simulink model "mrefrobotarm_modified_previous_y_previous_u_previous_ref_pert"  (R2018b)
settings: Solver=FixedStepAuto  StartTime=0.0  StopTime=10  RelTol=1e-3  AbsTol=1e-6
undefined symbols (not defined in the file or in its folder): cc, options
libraries: neural x714, simulink x1
(part 9 of 26)

== system mrefrobotarm_modified_previous_y_previous_u_previous_ref_pert/m=0.01 sd =0.01/Layer 3/Delays 1 ==
  "p{3}" : Inport  PortDimensions=30
      mask Display: e = 0.06;c1 = [120 230 180]/255;c2 = ([120 230 180]+0)/(256+128);c3 = ([120 230 180]+128)/(256+128);patch([0 1 1 0],[0 0 1 1],c1);patch([0 1 1 1-e 1-e 0+e],[0 0 1 1-e 0+e 0+e],c2);patch([0 0 1 1-e 0+e 0+e],[0 1 1 1-e 1-e 0+e],c3);plot([0 1 1 0 0],[0 0 1 1 0]);
  mux : Mux  Inputs=1
      mask Display: e = 0.06;c1 = [120 150 230]/255;c2 = ([120 150 230]+0)/383;c3 = ([120 150 230]+128)/383;patch([0 1 1 0],[0 0 1 1],c1);patch([0 1 1 1-e 1-e 0+e],[0 0 1 1-e 0+e 0+e],c2);patch([0 0 1 1-e 0+e 0+e],[0 1 1 1-e 1-e 0+e],c3);plot([0 1 1 0 0],[0 0 1 1 0]);disp('Mux')
  "pd{3,2}" : Outport
      mask Display: e = 0.06;c1 = [120 230 180]/255;c2 = ([120 230 180]+0)/(256+128);c3 = ([120 230 180]+128)/(256+128);patch([0 1 1 0],[0 0 1 1],c1);patch([0 1 1 1-e 1-e 0+e],[0 0 1 1-e 0+e 0+e],c2);patch([0 0 1 1-e 0+e 0+e],[0 1 1 1-e 1-e 0+e],c3);plot([0 1 1 0 0],[0 0 1 1 0]);
  wires:
  "p{3}"/1 -> mux/1
  mux/1 -> "pd{3,2}"/1

== system mrefrobotarm_modified_previous_y_previous_u_previous_ref_pert/m=0.01 sd =0.01/Layer 3/LW{3,2} ==
  "ad{3,2}" : Inport  PortDimensions=30
      mask Display: e = 0.06;c1 = [120 230 180]/255;c2 = ([120 230 180]+0)/(256+128);c3 = ([120 230 180]+128)/(256+128);patch([0 1 1 0],[0 0 1 1],c1);patch([0 1 1 1-e 1-e 0+e],[0 0 1 1-e 0+e 0+e],c2);patch([0 0 1 1-e 0+e 0+e],[0 1 1 1-e 1-e 0+e],c3);plot([0 1 1 0 0],[0 0 1 1 0]);
  "IW{3,2}(1,:)'" : Constant  Value=[0.0028381381201219024745796559727750718593597412109375;-0.00708260609535531389380214051243456196971237659454345703125;-0.00583488335220346855669593111315407440997660160064697265625;0.01020530930108067869943599959015045897103846073150634765625;0.0035026247420214058798937362126935113337822258472442626953125;0.007372665491954556553355626391521582263521850109100341796875;0.0082512842468972780185509918737807311117649078369140625;-0.006754245741655124334046345069282324402593076229095458984375;0.001683452101721956591096063249324288335628807544708251953125;-0.00690829099421421365112561119303791201673448085784912109375;0.01314880348478297822367721892078407108783721923828125;-0.007470263091506845927469715462621024926193058490753173828125;-0.00542419932097103381363201179965471965260803699493408203125;-0.01146260049752216743368382623202705872245132923126220703125;-0.009116602607925426704493787610772415064275264739990234375;-0.0032803912590090062058323372440327148069627583026885986328125;-0.006661633151908582205213971150215002126060426235198974609375;-0.0289839272926558366716420778175233863294124603271484375;0.007080157965975715332607176577539576101116836071014404296875;1.106395796742202453089021219057030975818634033203125;0.0098157682894019597508172836342055234126746654510498046875;-0.00914110666628639191577665457089096889831125736236572265625;-0.00060787204210546621867272687467220748658291995525360107421875;-0.00883143986489790498717322719812727882526814937591552734375;0.0082676478536601351321255748416660935617983341217041015625;-0.00932936505581516591079083156046181102283298969268798828125;-0.00127195106162408637373584241458956967107951641082763671875;-0.00692592170297301294723535391995028476230800151824951171875;0.009542106880190574791367197349245543591678142547607421875;-0.00879287702148130560775296515885202097706496715545654296875]
      mask Display: e = 0.06;c1 = [120 150 230]/255;c2 = ([120 150 230]+0)/383;c3 = ([120 150 230]+128)/383;patch([0 1 1 0],[0 0 1 1],c1);patch([0 1 1 1-e 1-e 0+e],[0 0 1 1-e 0+e 0+e],c2);patch([0 0 1 1-e 0+e 0+e],[0 1 1 1-e 1-e 0+e],c3);plot([0 1 1 0 0],[0 0 1 1 0]);disp('weights');
  Mux : Mux  Inputs=1
      mask Display: e = 0.06;c1 = [120 150 230]/255;c2 = ([120 150 230]+0)/383;c3 = ([120 150 230]+128)/383;patch([0 1 1 0],[0 0 1 1],c1);patch([0 1 1 1-e 1-e 0+e],[0 0 1 1-e 0+e 0+e],c2);patch([0 0 1 1-e 0+e 0+e],[0 1 1 1-e 1-e 0+e],c3);plot([0 1 1 0 0],[0 0 1 1 0]);disp('Mux');
  dotprod1 : neural/Weight Functions/dotprod
  "lz{3,2}" : Outport
      mask Display: e = 0.06;c1 = [120 230 180]/255;c2 = ([120 230 180]+0)/(256+128);c3 = ([120 230 180]+128)/(256+128);patch([0 1 1 0],[0 0 1 1],c1);patch([0 1 1 1-e 1-e 0+e],[0 0 1 1-e 0+e 0+e],c2);patch([0 0 1 1-e 0+e 0+e],[0 1 1 1-e 1-e 0+e],c3);plot([0 1 1 0 0],[0 0 1 1 0]);
  wires:
  "IW{3,2}(1,:)'"/1 -> dotprod1/1
  "ad{3,2}"/1 -> dotprod1/2
  dotprod1/1 -> Mux/1
  Mux/1 -> "lz{3,2}"/1

== system mrefrobotarm_modified_previous_y_previous_u_previous_ref_pert/m=0.01 sd=0.001/Layer 1/Delays 1 ==
  "p{1}" : Inport  PortDimensions=10
      mask Display: e = 0.06;c1 = [120 230 180]/255;c2 = ([120 230 180]+0)/(256+128);c3 = ([120 230 180]+128)/(256+128);patch([0 1 1 0],[0 0 1 1],c1);patch([0 1 1 1-e 1-e 0+e],[0 0 1 1-e 0+e 0+e],c2);patch([0 0 1 1-e 0+e 0+e],[0 1 1 1-e 1-e 0+e],c3);plot([0 1 1 0 0],[0 0 1 1 0]);
  mux : Mux  Inputs=1
      mask Display: e = 0.06;c1 = [120 150 230]/255;c2 = ([120 150 230]+0)/383;c3 = ([120 150 230]+128)/383;patch([0 1 1 0],[0 0 1 1],c1);patch([0 1 1 1-e 1-e 0+e],[0 0 1 1-e 0+e 0+e],c2);patch([0 0 1 1-e 0+e 0+e],[0 1 1 1-e 1-e 0+e],c3);plot([0 1 1 0 0],[0 0 1 1 0]);disp('Mux')
  "pd{1,1}" : Outport
      mask Display: e = 0.06;c1 = [120 230 180]/255;c2 = ([120 230 180]+0)/(256+128);c3 = ([120 230 180]+128)/(256+128);patch([0 1 1 0],[0 0 1 1],c1);patch([0 1 1 1-e 1-e 0+e],[0 0 1 1-e 0+e 0+e],c2);patch([0 0 1 1-e 0+e 0+e],[0 1 1 1-e 1-e 0+e],c3);plot([0 1 1 0 0],[0 0 1 1 0]);
  wires:
  "p{1}"/1 -> mux/1
  mux/1 -> "pd{1,1}"/1

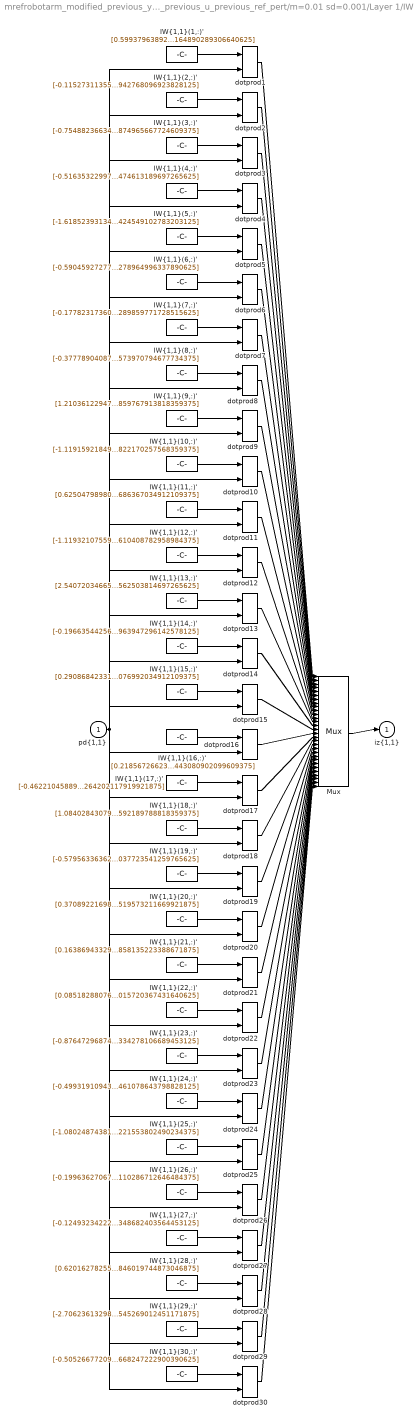
== system mrefrobotarm_modified_previous_y_previous_u_previous_ref_pert/m=0.01 sd=0.001/Layer 1/IW{1,1} ==
  "pd{1,1}" : Inport  PortDimensions=10
      mask Display: e = 0.06;c1 = [120 230 180]/255;c2 = ([120 230 180]+0)/(256+128);c3 = ([120 230 180]+128)/(256+128);patch([0 1 1 0],[0 0 1 1],c1);patch([0 1 1 1-e 1-e 0+e],[0 0 1 1-e 0+e 0+e],c2);patch([0 0 1 1-e 0+e 0+e],[0 1 1 1-e 1-e 0+e],c3);plot([0 1 1 0 0],[0 0 1 1 0]);
  "IW{1,1}(1,:)'" : Constant  Value=[0.59937963892562773349226290520164184272289276123046875;-0.396110549269906020430909165952471084892749786376953125;0.052609198895614932289799270392904873006045818328857421875;0.2316537316693900450115251032912055961787700653076171875;0.1524112985453686397452344181147054769098758697509765625;1.3349014602446771515786849704454652965068817138671875;-1.1072929840932717038270993725745938718318939208984375;0.5612431255418648401445125273312442004680633544921875;1.754962594866394720583002708735875785350799560546875;-0.7339839571900059755904521807678975164890289306640625]
      mask Display: e = 0.06;c1 = [120 150 230]/255;c2 = ([120 150 230]+0)/383;c3 = ([120 150 230]+128)/383;patch([0 1 1 0],[0 0 1 1],c1);patch([0 1 1 1-e 1-e 0+e],[0 0 1 1-e 0+e 0+e],c2);patch([0 0 1 1-e 0+e 0+e],[0 1 1 1-e 1-e 0+e],c3);plot([0 1 1 0 0],[0 0 1 1 0]);disp('Weights');
  "IW{1,1}(10,:)'" : Constant  Value=[-1.1191592184986463021090230540721677243709564208984375;0.486437593586613148399777628583251498639583587646484375;-0.2381955774681704662842918196474784053862094879150390625;-0.1603252511560420423553097180047188885509967803955078125;0.7021448810400536810760740991099737584590911865234375;-0.3126747431395717757851571150240488350391387939453125;0.53741683902639980630056015797890722751617431640625;0.79780181908275016322562578352517448365688323974609375;-0.364527373296976653360701448036707006394863128662109375;-0.7996723179317937191257215090445242822170257568359375]
      mask Display: e = 0.06;c1 = [120 150 230]/255;c2 = ([120 150 230]+0)/383;c3 = ([120 150 230]+128)/383;patch([0 1 1 0],[0 0 1 1],c1);patch([0 1 1 1-e 1-e 0+e],[0 0 1 1-e 0+e 0+e],c2);patch([0 0 1 1-e 0+e 0+e],[0 1 1 1-e 1-e 0+e],c3);plot([0 1 1 0 0],[0 0 1 1 0]);disp('Weights');
  "IW{1,1}(11,:)'" : Constant  Value=[0.62504798980455367196640281690633855760097503662109375;-0.408031907962375317566738885943777859210968017578125;0.501373014961266516564819539780728518962860107421875;0.4833802699139095881974981239181943237781524658203125;-0.362522530256057018416271375826909206807613372802734375;0.2813521372804477227447250697878189384937286376953125;0.8862870179180950547248585280613042414188385009765625;-1.4633494351540063949101977414102293550968170166015625;-0.8590052367755502960022795377881266176700592041015625;0.136037007850934477115600884644663892686367034912109375]
      mask Display: e = 0.06;c1 = [120 150 230]/255;c2 = ([120 150 230]+0)/383;c3 = ([120 150 230]+128)/383;patch([0 1 1 0],[0 0 1 1],c1);patch([0 1 1 1-e 1-e 0+e],[0 0 1 1-e 0+e 0+e],c2);patch([0 0 1 1-e 0+e 0+e],[0 1 1 1-e 1-e 0+e],c3);plot([0 1 1 0 0],[0 0 1 1 0]);disp('Weights');
  "IW{1,1}(12,:)'" : Constant  Value=[-1.119321075598907366810408348101191222667694091796875;-0.171441423142051962980048074314254336059093475341796875;0.980850911593684759992584076826460659503936767578125;0.3269671045177842128026668433449231088161468505859375;0.53034563893542718826523696407093666493892669677734375;-0.54427113197092236163143752492032945156097412109375;-0.74693143368845282825674303239793516695499420166015625;0.1287694280211927055912468631504452787339687347412109375;1.6486561129395822522525349995703436434268951416015625;1.0686346905333097279111598254530690610408782958984375]
      mask Display: e = 0.06;c1 = [120 150 230]/255;c2 = ([120 150 230]+0)/383;c3 = ([120 150 230]+128)/383;patch([0 1 1 0],[0 0 1 1],c1);patch([0 1 1 1-e 1-e 0+e],[0 0 1 1-e 0+e 0+e],c2);patch([0 0 1 1-e 0+e 0+e],[0 1 1 1-e 1-e 0+e],c3);plot([0 1 1 0 0],[0 0 1 1 0]);disp('Weights');
  "IW{1,1}(13,:)'" : Constant  Value=[2.5407203466529697521991693065501749515533447265625;-2.261223662409907131376485267537645995616912841796875;-0.365069530662350316685405005046050064265727996826171875;-0.1886766043105331525087109412197605706751346588134765625;0.0417142901719788350423101519481861032545566558837890625;0.480779756856362094907808568677864968776702880859375;-0.8817579284910894710236561877536587417125701904296875;0.0282120041976467554600827014610331389121711254119873046875;-1.2812114145188753244752888349466957151889801025390625;0.76789716007406616515851283111260272562503814697265625]
      mask Display: e = 0.06;c1 = [120 150 230]/255;c2 = ([120 150 230]+0)/383;c3 = ([120 150 230]+128)/383;patch([0 1 1 0],[0 0 1 1],c1);patch([0 1 1 1-e 1-e 0+e],[0 0 1 1-e 0+e 0+e],c2);patch([0 0 1 1-e 0+e 0+e],[0 1 1 1-e 1-e 0+e],c3);plot([0 1 1 0 0],[0 0 1 1 0]);disp('Weights');
  "IW{1,1}(14,:)'" : Constant  Value=[-0.196635442564636775397701740075717680156230926513671875;0.753137183083409933459506646613590419292449951171875;-0.5846087516227012059744083671830594539642333984375;0.0066653128689167229214973531270516104996204376220703125;0.87919069192101118037641072078258730471134185791015625;-1.478285060894569458156411201343871653079986572265625;1.056716341117762691936832197825424373149871826171875;-0.35476868904702529849970460418262518942356109619140625;-0.5897637965049866703992620386998169124126434326171875;-1.2665284785016901469845151950721628963947296142578125]
      mask Display: e = 0.06;c1 = [120 150 230]/255;c2 = ([120 150 230]+0)/383;c3 = ([120 150 230]+128)/383;patch([0 1 1 0],[0 0 1 1],c1);patch([0 1 1 1-e 1-e 0+e],[0 0 1 1-e 0+e 0+e],c2);patch([0 0 1 1-e 0+e 0+e],[0 1 1 1-e 1-e 0+e],c3);plot([0 1 1 0 0],[0 0 1 1 0]);disp('Weights');
  "IW{1,1}(15,:)'" : Constant  Value=[0.290868423311764157102032868351670913398265838623046875;-1.750593224807010184207456404692493379116058349609375;0.8684408095532607507749389696982689201831817626953125;0.369224320598639355051062693746644072234630584716796875;4.0877592364522090662148912088014185428619384765625;-1.7860833750709534939460354507900774478912353515625;0.274764925669300497101943392408429645001888275146484375;-0.290579497554917853818778894492425024509429931640625;-0.907612828107296376600743315066210925579071044921875;0.046258718737966962597507603049962199293076992034912109375]
      mask Display: e = 0.06;c1 = [120 150 230]/255;c2 = ([120 150 230]+0)/383;c3 = ([120 150 230]+128)/383;patch([0 1 1 0],[0 0 1 1],c1);patch([0 1 1 1-e 1-e 0+e],[0 0 1 1-e 0+e 0+e],c2);patch([0 0 1 1-e 0+e 0+e],[0 1 1 1-e 1-e 0+e],c3);plot([0 1 1 0 0],[0 0 1 1 0]);disp('Weights');
  "IW{1,1}(16,:)'" : Constant  Value=[0.21856726623393207820100769822602160274982452392578125;0.43822988527784667578401922582997940480709075927734375;-0.139288002716730641150633118741097860038280487060546875;0.47802454669038885182175135923898778855800628662109375;-2.458877629721705648790930354152806103229522705078125;0.73280849029216710288636704717646352946758270263671875;0.279458397030770300251134585778345353901386260986328125;0.62598650250979093190295543536194600164890289306640625;1.01423895682535913920219172723591327667236328125;-0.173414588391354873575522788087255321443080902099609375]
      mask Display: e = 0.06;c1 = [120 150 230]/255;c2 = ([120 150 230]+0)/383;c3 = ([120 150 230]+128)/383;patch([0 1 1 0],[0 0 1 1],c1);patch([0 1 1 1-e 1-e 0+e],[0 0 1 1-e 0+e 0+e],c2);patch([0 0 1 1-e 0+e 0+e],[0 1 1 1-e 1-e 0+e],c3);plot([0 1 1 0 0],[0 0 1 1 0]);disp('Weights');
  "IW{1,1}(17,:)'" : Constant  Value=[-0.462210458898908715941189484510687179863452911376953125;0.0562441048399441589911162964199320413172245025634765625;1.6557581521501216759162389280390925705432891845703125;1.4468927892442950966511716615059413015842437744140625;-0.404186313250386841655625858038547448813915252685546875;0.271837747395356765789387054610415361821651458740234375;-1.263092687688632143050426748231984674930572509765625;0.185960700398180633907685432859580032527446746826171875;2.02659382751513650333663463243283331394195556640625;-0.40086308697406003442864630414987914264202117919921875]
      mask Display: e = 0.06;c1 = [120 150 230]/255;c2 = ([120 150 230]+0)/383;c3 = ([120 150 230]+128)/383;patch([0 1 1 0],[0 0 1 1],c1);patch([0 1 1 1-e 1-e 0+e],[0 0 1 1-e 0+e 0+e],c2);patch([0 0 1 1-e 0+e 0+e],[0 1 1 1-e 1-e 0+e],c3);plot([0 1 1 0 0],[0 0 1 1 0]);disp('Weights');
  "IW{1,1}(18,:)'" : Constant  Value=[1.0840284307910679206798931772937066853046417236328125;0.04238645655672386436396692488415283150970935821533203125;0.0647929422435409296809893930912949144840240478515625;-0.2007261202465783489490291913170949555933475494384765625;0.231390749330992295806908032318460755050182342529296875;-0.2493164861823878031277246236641076393425464630126953125;-1.288247138719182061095125391148030757904052734375;0.66489830287387075014038373410585336387157440185546875;-0.87855236053860064071585611600312404334545135498046875;-0.571013622141661070230611585429869592189788818359375]
      mask Display: e = 0.06;c1 = [120 150 230]/255;c2 = ([120 150 230]+0)/383;c3 = ([120 150 230]+128)/383;patch([0 1 1 0],[0 0 1 1],c1);patch([0 1 1 1-e 1-e 0+e],[0 0 1 1-e 0+e 0+e],c2);patch([0 0 1 1-e 0+e 0+e],[0 1 1 1-e 1-e 0+e],c3);plot([0 1 1 0 0],[0 0 1 1 0]);disp('Weights');
  "IW{1,1}(19,:)'" : Constant  Value=[-0.579563363622992877566275637946091592311859130859375;0.0808814352621067544912847324667382054030895233154296875;-0.627693531991440512030067111481912434101104736328125;-0.342503079851861347293606741004623472690582275390625;1.9480020511887434775388783236849121749401092529296875;-1.22709210487031139535929469275288283824920654296875;-1.041532997170801166930687031708657741546630859375;-0.40601996839724840970831110098515637218952178955078125;-0.350497880443465359423527161197853274643421173095703125;0.379106573287681547501648537945584394037723541259765625]
      mask Display: e = 0.06;c1 = [120 150 230]/255;c2 = ([120 150 230]+0)/383;c3 = ([120 150 230]+128)/383;patch([0 1 1 0],[0 0 1 1],c1);patch([0 1 1 1-e 1-e 0+e],[0 0 1 1-e 0+e 0+e],c2);patch([0 0 1 1-e 0+e 0+e],[0 1 1 1-e 1-e 0+e],c3);plot([0 1 1 0 0],[0 0 1 1 0]);disp('Weights');
  "IW{1,1}(2,:)'" : Constant  Value=[-0.11527311355962044370215835442650131881237030029296875;-0.404225992456426597154717228477238677442073822021484375;-0.334837070807286918405765163697651587426662445068359375;0.90518533001313794539299806274357251822948455810546875;2.2543779617530912418033040012232959270477294921875;-2.026726348690087053938668759656138718128204345703125;-0.21181078080885329395499638849287293851375579833984375;-1.79130234483826011882001694175414741039276123046875;1.1268087142547169587913913346710614860057830810546875;-0.97828729118855151103417711055953986942768096923828125]
      mask Display: e = 0.06;c1 = [120 150 230]/255;c2 = ([120 150 230]+0)/383;c3 = ([120 150 230]+128)/383;patch([0 1 1 0],[0 0 1 1],c1);patch([0 1 1 1-e 1-e 0+e],[0 0 1 1-e 0+e 0+e],c2);patch([0 0 1 1-e 0+e 0+e],[0 1 1 1-e 1-e 0+e],c3);plot([0 1 1 0 0],[0 0 1 1 0]);disp('Weights');
  "IW{1,1}(20,:)'" : Constant  Value=[0.370892216980794497960260969193768687546253204345703125;1.8302016509147744915964040046674199402332305908203125;-1.8556216709284181209937969470047391951084136962890625;1.655754682395713661691161178168840706348419189453125;-0.74706859881024545444461182341910898685455322265625;0.8604515450150509447979629840119741857051849365234375;-1.802061941623871010875745923840440809726715087890625;0.12266944769845385121431746711095911450684070587158203125;-2.192229171652474661868836847133934497833251953125;0.367378607338902873902242163239861838519573211669921875]
      mask Display: e = 0.06;c1 = [120 150 230]/255;c2 = ([120 150 230]+0)/383;c3 = ([120 150 230]+128)/383;patch([0 1 1 0],[0 0 1 1],c1);patch([0 1 1 1-e 1-e 0+e],[0 0 1 1-e 0+e 0+e],c2);patch([0 0 1 1-e 0+e 0+e],[0 1 1 1-e 1-e 0+e],c3);plot([0 1 1 0 0],[0 0 1 1 0]);disp('Weights');
  "IW{1,1}(21,:)'" : Constant  Value=[0.1638694332917713103459078638479695655405521392822265625;-0.302284193263745393220887081042747013270854949951171875;-0.385412062490031626094122430004063062369823455810546875;0.8129911212999463288042534259147942066192626953125;-0.85191701402662811659638464334420859813690185546875;-0.53939451890989664750719612129614688456058502197265625;0.441389074698777250649328607323695905506610870361328125;0.5769130466845950877541326917707920074462890625;-1.245667655438771337372827474609948694705963134765625;0.00412112726435204072827911403464895556680858135223388671875]
      mask Display: e = 0.06;c1 = [120 150 230]/255;c2 = ([120 150 230]+0)/383;c3 = ([120 150 230]+128)/383;patch([0 1 1 0],[0 0 1 1],c1);patch([0 1 1 1-e 1-e 0+e],[0 0 1 1-e 0+e 0+e],c2);patch([0 0 1 1-e 0+e 0+e],[0 1 1 1-e 1-e 0+e],c3);plot([0 1 1 0 0],[0 0 1 1 0]);disp('Weights');
  "IW{1,1}(22,:)'" : Constant  Value=[0.08518288076987053092370416607082006521522998809814453125;-0.8537294142013858166961881579481996595859527587890625;0.7741003486488844398394348900183103978633880615234375;0.158479487052409606651082185635459609329700469970703125;-1.6855139048679979030254116878495551645755767822265625;0.2147391184469020775082981344894506037235260009765625;-0.227385538868920378252624914239277131855487823486328125;-0.00452640259162017007110723199048152309842407703399658203125;0.9402929814598015578752665533102117478847503662109375;1.4362169500364247998192013255902566015720367431640625]
      mask Display: e = 0.06;c1 = [120 150 230]/255;c2 = ([120 150 230]+0)/383;c3 = ([120 150 230]+128)/383;patch([0 1 1 0],[0 0 1 1],c1);patch([0 1 1 1-e 1-e 0+e],[0 0 1 1-e 0+e 0+e],c2);patch([0 0 1 1-e 0+e 0+e],[0 1 1 1-e 1-e 0+e],c3);plot([0 1 1 0 0],[0 0 1 1 0]);disp('Weights');
  "IW{1,1}(23,:)'" : Constant  Value=[-0.876472968740060753845000363071449100971221923828125;0.97338759015756204373559512532665394246578216552734375;0.048119337681629716085840442474363953806459903717041015625;0.041438003349266304409237449135616770945489406585693359375;-0.126305138511878689566714228931232355535030364990234375;1.00882944072944980007378035224974155426025390625;-0.93544391369868529206854645963176153600215911865234375;-0.2308533783162892427665013883597566746175289154052734375;-1.6617951684667169320874791083042509853839874267578125;0.07859271650706974032818408204548177309334278106689453125]
      mask Display: e = 0.06;c1 = [120 150 230]/255;c2 = ([120 150 230]+0)/383;c3 = ([120 150 230]+128)/383;patch([0 1 1 0],[0 0 1 1],c1);patch([0 1 1 1-e 1-e 0+e],[0 0 1 1-e 0+e 0+e],c2);patch([0 0 1 1-e 0+e 0+e],[0 1 1 1-e 1-e 0+e],c3);plot([0 1 1 0 0],[0 0 1 1 0]);disp('Weights');
  "IW{1,1}(24,:)'" : Constant  Value=[-0.499319109438899733088845778183895163238048553466796875;0.0249813223099573898655645365352029330097138881683349609375;-0.62391102764310557571292292777798138558864593505859375;0.045969549982219193307031446238397620618343353271484375;0.29761373371729582526512558615650050342082977294921875;0.75652230673170783870062905407394282519817352294921875;-0.21882391321545358042754969574161805212497711181640625;-0.152652868546594489007617312381626106798648834228515625;0.130026205414276230243331156088970601558685302734375;0.210042947632892051945674438684363849461078643798828125]
      mask Display: e = 0.06;c1 = [120 150 230]/255;c2 = ([120 150 230]+0)/383;c3 = ([120 150 230]+128)/383;patch([0 1 1 0],[0 0 1 1],c1);patch([0 1 1 1-e 1-e 0+e],[0 0 1 1-e 0+e 0+e],c2);patch([0 0 1 1-e 0+e 0+e],[0 1 1 1-e 1-e 0+e],c3);plot([0 1 1 0 0],[0 0 1 1 0]);disp('Weights');
  "IW{1,1}(25,:)'" : Constant  Value=[-1.080248743819219203743386970018036663532257080078125;0.90199303598355073940950887845247052609920501708984375;-0.81531722448001942016304610660881735384464263916015625;-0.470572048901045481006377713129040785133838653564453125;-0.215494082328827440964147399427019990980625152587890625;0.73105039783397585129165463513345457613468170166015625;-2.073647250650516138392731591011397540569305419921875;0.0858309743410513303896181014351896010339260101318359375;0.22192825146346584208600916099385358393192291259765625;0.20410220428678493842511443290277384221553802490234375]
      mask Display: e = 0.06;c1 = [120 150 230]/255;c2 = ([120 150 230]+0)/383;c3 = ([120 150 230]+128)/383;patch([0 1 1 0],[0 0 1 1],c1);patch([0 1 1 1-e 1-e 0+e],[0 0 1 1-e 0+e 0+e],c2);patch([0 0 1 1-e 0+e 0+e],[0 1 1 1-e 1-e 0+e],c3);plot([0 1 1 0 0],[0 0 1 1 0]);disp('Weights');
  "IW{1,1}(26,:)'" : Constant  Value=[-0.199636270672255478064727185483206994831562042236328125;0.466242803891780577263403984034084714949131011962890625;-1.786751590761676222740561570390127599239349365234375;0.00230779769893033580296926032815463258884847164154052734375;1.2852038464398283235112785405362956225872039794921875;-1.0973774958082704866768608553684316575527191162109375;0.308005670144092358331278092009597457945346832275390625;-0.35227734504899654854881418941658921539783477783203125;1.0752875894278357549183056107722222805023193359375;-0.38697375163509251105864450437366031110286712646484375]
      mask Display: e = 0.06;c1 = [120 150 230]/255;c2 = ([120 150 230]+0)/383;c3 = ([120 150 230]+128)/383;patch([0 1 1 0],[0 0 1 1],c1);patch([0 1 1 1-e 1-e 0+e],[0 0 1 1-e 0+e 0+e],c2);patch([0 0 1 1-e 0+e 0+e],[0 1 1 1-e 1-e 0+e],c3);plot([0 1 1 0 0],[0 0 1 1 0]);disp('Weights');
  "IW{1,1}(27,:)'" : Constant  Value=[-0.124932342227794979105937045460450462996959686279296875;-0.66631572445832720763547740716603584587574005126953125;-0.02202657447860668915584625437986687757074832916259765625;-0.1792737902950718720251899185313959605991840362548828125;0.4624051360576657554446455833385698497295379638671875;-0.048505735738689235991838444306267774663865566253662109375;0.269052190115036282680449630788643844425678253173828125;0.1233902147738448196179206206579692661762237548828125;0.145988756281055953589742557596764527261257171630859375;0.82365531327662655503019095704075880348682403564453125]
      mask Display: e = 0.06;c1 = [120 150 230]/255;c2 = ([120 150 230]+0)/383;c3 = ([120 150 230]+128)/383;patch([0 1 1 0],[0 0 1 1],c1);patch([0 1 1 1-e 1-e 0+e],[0 0 1 1-e 0+e 0+e],c2);patch([0 0 1 1-e 0+e 0+e],[0 1 1 1-e 1-e 0+e],c3);plot([0 1 1 0 0],[0 0 1 1 0]);disp('Weights');
  "IW{1,1}(28,:)'" : Constant  Value=[0.62016278255009071873615766889997757971286773681640625;0.03190241625757568588728219083350268192589282989501953125;-0.544385606509863340107813201029784977436065673828125;0.1453635890249763418236028655883274041116237640380859375;-0.60065937150521875320663411912391893565654754638671875;-1.1049035559021211927444028333411552011966705322265625;0.312613407122662056991657664184458553791046142578125;0.5588976319380625223942615775740705430507659912109375;-0.93021207078281531455132835617405362427234649658203125;0.74350140785050367053798936467501334846019744873046875]
      mask Display: e = 0.06;c1 = [120 150 230]/255;c2 = ([120 150 230]+0)/383;c3 = ([120 150 230]+128)/383;patch([0 1 1 0],[0 0 1 1],c1);patch([0 1 1 1-e 1-e 0+e],[0 0 1 1-e 0+e 0+e],c2);patch([0 0 1 1-e 0+e 0+e],[0 1 1 1-e 1-e 0+e],c3);plot([0 1 1 0 0],[0 0 1 1 0]);disp('Weights');
  "IW{1,1}(29,:)'" : Constant  Value=[-2.706236132987961173768098888103850185871124267578125;1.605665021864861596867513071629218757152557373046875;0.526580609549972766814107671962119638919830322265625;-0.14272486709085985268075091880746185779571533203125;-1.312819169084094905741721959202550351619720458984375;1.147345692737551825501896018977276980876922607421875;0.410746459531053986768966979070683009922504425048828125;1.2852081431608881612049799514352343976497650146484375;0.1081836722584629539856138080722303129732608795166015625;0.73857624379430841798921392182819545269012451171875]
      mask Display: e = 0.06;c1 = [120 150 230]/255;c2 = ([120 150 230]+0)/383;c3 = ([120 150 230]+128)/383;patch([0 1 1 0],[0 0 1 1],c1);patch([0 1 1 1-e 1-e 0+e],[0 0 1 1-e 0+e 0+e],c2);patch([0 0 1 1-e 0+e 0+e],[0 1 1 1-e 1-e 0+e],c3);plot([0 1 1 0 0],[0 0 1 1 0]);disp('Weights');
  "IW{1,1}(3,:)'" : Constant  Value=[-0.75488236634097571897683565111947245895862579345703125;0.3670412473066251290987338506965897977352142333984375;1.01240774526453236603629193268716335296630859375;0.7161619255534501515825240858248434960842132568359375;0.25623477060716293163267209820332936942577362060546875;1.580258141643140046284088384709320962429046630859375;-0.288265922013249298316850399714894592761993408203125;-0.042314819711078734132403411649647750891745090484619140625;0.5350196659118566788748694307287223637104034423828125;0.3356458871309120350900911944336257874965667724609375]
      mask Display: e = 0.06;c1 = [120 150 230]/255;c2 = ([120 150 230]+0)/383;c3 = ([120 150 230]+128)/383;patch([0 1 1 0],[0 0 1 1],c1);patch([0 1 1 1-e 1-e 0+e],[0 0 1 1-e 0+e 0+e],c2);patch([0 0 1 1-e 0+e 0+e],[0 1 1 1-e 1-e 0+e],c3);plot([0 1 1 0 0],[0 0 1 1 0]);disp('Weights');
  "IW{1,1}(30,:)'" : Constant  Value=[-0.50526677209464765372359806860913522541522979736328125;-0.7086058290307359897042260854505002498626708984375;0.80288187329153604121501075496780686080455780029296875;0.3084326872686131704170975353918038308620452880859375;0.011191847348981577570103951302371569909155368804931640625;-0.13027295381265435736395374988205730915069580078125;-0.63120307203300252130162562025361694395542144775390625;0.59429072606559441016571554428082890808582305908203125;0.98981309673762296608146016296814195811748504638671875;-0.0754501604676642845248579760664142668247222900390625]
      mask Display: e = 0.06;c1 = [120 150 230]/255;c2 = ([120 150 230]+0)/383;c3 = ([120 150 230]+128)/383;patch([0 1 1 0],[0 0 1 1],c1);patch([0 1 1 1-e 1-e 0+e],[0 0 1 1-e 0+e 0+e],c2);patch([0 0 1 1-e 0+e 0+e],[0 1 1 1-e 1-e 0+e],c3);plot([0 1 1 0 0],[0 0 1 1 0]);disp('Weights');
  "IW{1,1}(4,:)'" : Constant  Value=[-0.516353229978596228733067619032226502895355224609375;-1.103631081466493579767984556383453309535980224609375;0.7578291006076636193711237865500152111053466796875;-0.482376012038346624333229328840388916432857513427734375;-1.4371596262453063541641995470854453742504119873046875;-0.1944939411233803927547825196597841568291187286376953125;1.56897655385656431548113687313161790370941162109375;1.288771842824615987410652451217174530029296875;0.0142198876681832973856156598913003108464181423187255859375;0.2646892221021150959359147236682474613189697265625]
      mask Display: e = 0.06;c1 = [120 150 230]/255;c2 = ([120 150 230]+0)/383;c3 = ([120 150 230]+128)/383;patch([0 1 1 0],[0 0 1 1],c1);patch([0 1 1 1-e 1-e 0+e],[0 0 1 1-e 0+e 0+e],c2);patch([0 0 1 1-e 0+e 0+e],[0 1 1 1-e 1-e 0+e],c3);plot([0 1 1 0 0],[0 0 1 1 0]);disp('Weights');
  "IW{1,1}(5,:)'" : Constant  Value=[-1.6185239313409771622076505082077346742153167724609375;0.66121160958456537404259734103106893599033355712890625;0.49893121833904652273616875390871427953243255615234375;-0.0022013083249246136012533536785440446692518889904022216796875;0.33840270003378714047670428044511936604976654052734375;1.8341241878053580194318783469498157501220703125;-1.4131691826434986669625004651607014238834381103515625;0.31651863826449588845690641392138786613941192626953125;0.83507561497049509480206097578047774732112884521484375;-0.2197673461643170622625831356344860978424549102783203125]
      mask Display: e = 0.06;c1 = [120 150 230]/255;c2 = ([120 150 230]+0)/383;c3 = ([120 150 230]+128)/383;patch([0 1 1 0],[0 0 1 1],c1);patch([0 1 1 1-e 1-e 0+e],[0 0 1 1-e 0+e 0+e],c2);patch([0 0 1 1-e 0+e 0+e],[0 1 1 1-e 1-e 0+e],c3);plot([0 1 1 0 0],[0 0 1 1 0]);disp('Weights');
  "IW{1,1}(6,:)'" : Constant  Value=[-0.590459272773774745957098275539465248584747314453125;0.55052745113397139054001172553398646414279937744140625;-0.81263114027772653802372815334820188581943511962890625;-0.43956190723335686332262639552936889231204986572265625;-1.973825194590407949846166957286186516284942626953125;2.03599524499412698474998251185752451419830322265625;-0.335927600637568268826527173587237484753131866455078125;-0.804229659678409536383014710736460983753204345703125;0.0809369564142785602456342530786059796810150146484375;1.1115959245337629912597776637994684278964996337890625]
      mask Display: e = 0.06;c1 = [120 150 230]/255;c2 = ([120 150 230]+0)/383;c3 = ([120 150 230]+128)/383;patch([0 1 1 0],[0 0 1 1],c1);patch([0 1 1 1-e 1-e 0+e],[0 0 1 1-e 0+e 0+e],c2);patch([0 0 1 1-e 0+e 0+e],[0 1 1 1-e 1-e 0+e],c3);plot([0 1 1 0 0],[0 0 1 1 0]);disp('Weights');
  "IW{1,1}(7,:)'" : Constant  Value=[-0.177823173605108630912496892051422037184238433837890625;-0.1643050204328404817477604638042976148426532745361328125;-0.66501256984892875845361004394362680613994598388671875;0.65392664211458717549163566218339838087558746337890625;-1.3627966765753674049932442358112893998622894287109375;0.60552086375707403487211877290974371135234832763671875;0.1617097296379933213383850443278788588941097259521484375;-0.7858432318438748342970256999251432716846466064453125;-0.285345159763251421392027395995683036744594573974609375;-1.1360349772904767551295890370965935289859771728515625]
      mask Display: e = 0.06;c1 = [120 150 230]/255;c2 = ([120 150 230]+0)/383;c3 = ([120 150 230]+128)/383;patch([0 1 1 0],[0 0 1 1],c1);patch([0 1 1 1-e 1-e 0+e],[0 0 1 1-e 0+e 0+e],c2);patch([0 0 1 1-e 0+e 0+e],[0 1 1 1-e 1-e 0+e],c3);plot([0 1 1 0 0],[0 0 1 1 0]);disp('Weights');
  "IW{1,1}(8,:)'" : Constant  Value=[-0.3777890408735229410552847184590063989162445068359375;0.199557963606572796866345242960960604250431060791015625;-1.0658180942259518619863456478924490511417388916015625;-0.58240836266738182924740385715267620980739593505859375;1.9240505212844880578160200457205064594745635986328125;-0.150131019153114220188172112102620303630828857421875;-0.69003600114381213881387111541698686778545379638671875;-2.317590874130956990484264679253101348876953125;-1.07442710253165341072190130944363772869110107421875;0.88066878297068507119860214515938423573970794677734375]
      mask Display: e = 0.06;c1 = [120 150 230]/255;c2 = ([120 150 230]+0)/383;c3 = ([120 150 230]+128)/383;patch([0 1 1 0],[0 0 1 1],c1);patch([0 1 1 1-e 1-e 0+e],[0 0 1 1-e 0+e 0+e],c2);patch([0 0 1 1-e 0+e 0+e],[0 1 1 1-e 1-e 0+e],c3);plot([0 1 1 0 0],[0 0 1 1 0]);disp('Weights');
  "IW{1,1}(9,:)'" : Constant  Value=[1.210361229471092148202160387882031500339508056640625;-0.68513372757470225593579016276635229587554931640625;-1.1011702829165497252716932052862830460071563720703125;0.356373372111487174418442691603559069335460662841796875;2.116302407247494077324745376245118677616119384765625;-1.141129897723512254259503606590442359447479248046875;-0.1456365482338088657154884231204050593078136444091796875;0.40462029499123841613794638760737143456935882568359375;0.247603059472719488898206918747746385633945465087890625;1.5065691403281105120726124368957243859767913818359375]
      mask Display: e = 0.06;c1 = [120 150 230]/255;c2 = ([120 150 230]+0)/383;c3 = ([120 150 230]+128)/383;patch([0 1 1 0],[0 0 1 1],c1);patch([0 1 1 1-e 1-e 0+e],[0 0 1 1-e 0+e 0+e],c2);patch([0 0 1 1-e 0+e 0+e],[0 1 1 1-e 1-e 0+e],c3);plot([0 1 1 0 0],[0 0 1 1 0]);disp('Weights');
  Mux : Mux  Inputs=30
      mask Display: e = 0.06;c1 = [120 150 230]/255;c2 = ([120 150 230]+0)/383;c3 = ([120 150 230]+128)/383;patch([0 1 1 0],[0 0 1 1],c1);patch([0 1 1 1-e 1-e 0+e],[0 0 1 1-e 0+e 0+e],c2);patch([0 0 1 1-e 0+e 0+e],[0 1 1 1-e 1-e 0+e],c3);plot([0 1 1 0 0],[0 0 1 1 0]);disp('Mux');
  dotprod{1..30} (30 alike) : neural/Weight Functions/dotprod
  "iz{1,1}" : Outport
      mask Display: e = 0.06;c1 = [120 230 180]/255;c2 = ([120 230 180]+0)/(256+128);c3 = ([120 230 180]+128)/(256+128);patch([0 1 1 0],[0 0 1 1],c1);patch([0 1 1 1-e 1-e 0+e],[0 0 1 1-e 0+e 0+e],c2);patch([0 0 1 1-e 0+e 0+e],[0 1 1 1-e 1-e 0+e],c3);plot([0 1 1 0 0],[0 0 1 1 0]);
  wires:
  "IW{1,1}(1,:)'"/1 -> dotprod1/1
  "pd{1,1}"/1 -> dotprod1/2, dotprod2/2, dotprod3/2, dotprod4/2, dotprod5/2, dotprod6/2, dotprod7/2, dotprod8/2, dotprod9/2, dotprod10/2, dotprod11/2, dotprod12/2, dotprod13/2, dotprod14/2, dotprod15/2, dotprod16/2, dotprod17/2, dotprod18/2, dotprod19/2, dotprod20/2, dotprod21/2, dotprod22/2, dotprod23/2, dotprod24/2, dotprod25/2, dotprod26/2, dotprod27/2, dotprod28/2, dotprod29/2, dotprod30/2
  dotprod1/1 -> Mux/1
  "IW{1,1}(2,:)'"/1 -> dotprod2/1
  dotprod2/1 -> Mux/2
  "IW{1,1}(3,:)'"/1 -> dotprod3/1
  dotprod3/1 -> Mux/3
  "IW{1,1}(4,:)'"/1 -> dotprod4/1
  dotprod4/1 -> Mux/4
  "IW{1,1}(5,:)'"/1 -> dotprod5/1
  dotprod5/1 -> Mux/5
  "IW{1,1}(6,:)'"/1 -> dotprod6/1
  dotprod6/1 -> Mux/6
  "IW{1,1}(7,:)'"/1 -> dotprod7/1
  dotprod7/1 -> Mux/7
  "IW{1,1}(8,:)'"/1 -> dotprod8/1
  dotprod8/1 -> Mux/8
  "IW{1,1}(9,:)'"/1 -> dotprod9/1
  dotprod9/1 -> Mux/9
  "IW{1,1}(10,:)'"/1 -> dotprod10/1
  dotprod10/1 -> Mux/10
  "IW{1,1}(11,:)'"/1 -> dotprod11/1
  dotprod11/1 -> Mux/11
  "IW{1,1}(12,:)'"/1 -> dotprod12/1
  dotprod12/1 -> Mux/12
  "IW{1,1}(13,:)'"/1 -> dotprod13/1
  dotprod13/1 -> Mux/13
  "IW{1,1}(14,:)'"/1 -> dotprod14/1
  dotprod14/1 -> Mux/14
  "IW{1,1}(15,:)'"/1 -> dotprod15/1
  dotprod15/1 -> Mux/15
  "IW{1,1}(16,:)'"/1 -> dotprod16/1
  dotprod16/1 -> Mux/16
  "IW{1,1}(17,:)'"/1 -> dotprod17/1
  dotprod17/1 -> Mux/17
  "IW{1,1}(18,:)'"/1 -> dotprod18/1
  dotprod18/1 -> Mux/18
  "IW{1,1}(19,:)'"/1 -> dotprod19/1
  dotprod19/1 -> Mux/19
  "IW{1,1}(20,:)'"/1 -> dotprod20/1
  dotprod20/1 -> Mux/20
  "IW{1,1}(21,:)'"/1 -> dotprod21/1
  dotprod21/1 -> Mux/21
  "IW{1,1}(22,:)'"/1 -> dotprod22/1
  dotprod22/1 -> Mux/22
  "IW{1,1}(23,:)'"/1 -> dotprod23/1
  dotprod23/1 -> Mux/23
  "IW{1,1}(24,:)'"/1 -> dotprod24/1
  dotprod24/1 -> Mux/24
  "IW{1,1}(25,:)'"/1 -> dotprod25/1
  dotprod25/1 -> Mux/25
  "IW{1,1}(26,:)'"/1 -> dotprod26/1
  dotprod26/1 -> Mux/26
  "IW{1,1}(27,:)'"/1 -> dotprod27/1
  dotprod27/1 -> Mux/27
  "IW{1,1}(28,:)'"/1 -> dotprod28/1
  dotprod28/1 -> Mux/28
  "IW{1,1}(29,:)'"/1 -> dotprod29/1
  dotprod29/1 -> Mux/29
  "IW{1,1}(30,:)'"/1 -> dotprod30/1
  dotprod30/1 -> Mux/30
  Mux/1 -> "iz{1,1}"/1

== system mrefrobotarm_modified_previous_y_previous_u_previous_ref_pert/m=0.01 sd=0.001/Layer 2/Delays 1 ==
  "p{2}" : Inport  PortDimensions=30
      mask Display: e = 0.06;c1 = [120 230 180]/255;c2 = ([120 230 180]+0)/(256+128);c3 = ([120 230 180]+128)/(256+128);patch([0 1 1 0],[0 0 1 1],c1);patch([0 1 1 1-e 1-e 0+e],[0 0 1 1-e 0+e 0+e],c2);patch([0 0 1 1-e 0+e 0+e],[0 1 1 1-e 1-e 0+e],c3);plot([0 1 1 0 0],[0 0 1 1 0]);
  mux : Mux  Inputs=1
      mask Display: e = 0.06;c1 = [120 150 230]/255;c2 = ([120 150 230]+0)/383;c3 = ([120 150 230]+128)/383;patch([0 1 1 0],[0 0 1 1],c1);patch([0 1 1 1-e 1-e 0+e],[0 0 1 1-e 0+e 0+e],c2);patch([0 0 1 1-e 0+e 0+e],[0 1 1 1-e 1-e 0+e],c3);plot([0 1 1 0 0],[0 0 1 1 0]);disp('Mux')
  "pd{2,1}" : Outport
      mask Display: e = 0.06;c1 = [120 230 180]/255;c2 = ([120 230 180]+0)/(256+128);c3 = ([120 230 180]+128)/(256+128);patch([0 1 1 0],[0 0 1 1],c1);patch([0 1 1 1-e 1-e 0+e],[0 0 1 1-e 0+e 0+e],c2);patch([0 0 1 1-e 0+e 0+e],[0 1 1 1-e 1-e 0+e],c3);plot([0 1 1 0 0],[0 0 1 1 0]);
  wires:
  "p{2}"/1 -> mux/1
  mux/1 -> "pd{2,1}"/1
